simulink model "recovered_model"  (R2024b)
settings: Solver=VariableStepAuto  StartTime=0.0  StopTime=10.0  RelTol=1e-3
libraries: spsIGBTDiodeLib x4, spsSeriesRLCBranchLib x2, spsDCVoltageSourceLib x1, simulink x1, spsVoltageMeasurementLib x1, spspowerguiLib x1
settings Model: Creator=tiany  LastModifiedBy=tiany

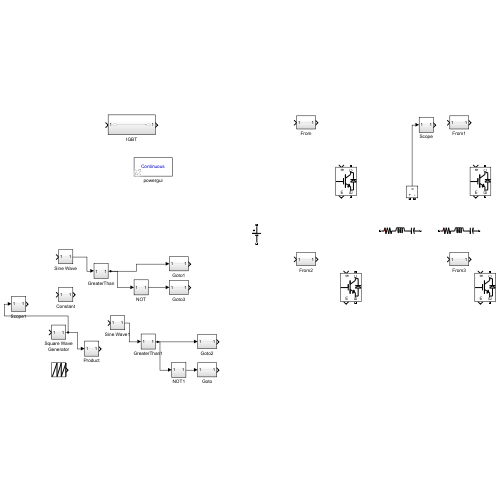
[thumbnail: Simulink's stored preview of the top-level diagram]
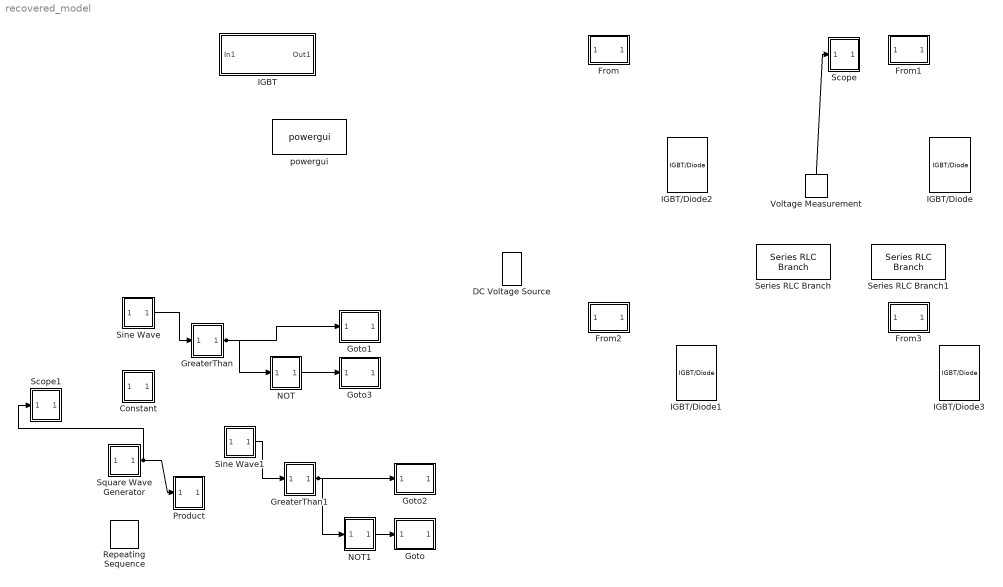
== system recovered_model ==
  Constant : Subsystem
  DC Voltage Source : spsDCVoltageSourceLib/DC Voltage Source  Amplitude=100  Measurements=None
  From : Subsystem
  From1 : Subsystem
  From2 : Subsystem
  From3 : Subsystem
  Goto : Subsystem
  Goto1 : Subsystem
  Goto2 : Subsystem
  Goto3 : Subsystem
  GreaterThan : Subsystem
  GreaterThan1 : Subsystem
  IGBT : Subsystem
  IGBT/Diode{,1..3} (4 alike) : spsIGBTDiodeLib/IGBT//Diode  Ron=1e-3  Rs=1e5  Cs=inf  Measurements=on
  NOT : Subsystem
  NOT1 : Subsystem
  Product : Subsystem
  Repeating Sequence : simulink/Sources/Repeating Sequence  rep_seq_t=[0 2]  rep_seq_y=[0 2]
  Scope : Subsystem
  Scope1 : Subsystem
  Series RLC Branch : spsSeriesRLCBranchLib/Series RLC Branch  LConnTagsString=__new0  RConnTagsString=__new0  BranchType=RLC  Resistance=1  Inductance=1e-3  SetiL0=off  InitialCurrent=0  Capacitance=1e-6  Setx0=off  InitialVoltage=0  Measurements=None
  Series RLC Branch1 : spsSeriesRLCBranchLib/Series RLC Branch  LConnTagsString=__new0  RConnTagsString=__new0  BranchType=RLC  Resistance=1  Inductance=1e-3  SetiL0=off  InitialCurrent=0  Capacitance=1e-6  Setx0=off  InitialVoltage=0  Measurements=None
  Sine Wave : Subsystem
  Sine Wave1 : Subsystem
  Square Wave Generator : Subsystem
  Voltage Measurement : spsVoltageMeasurementLib/Voltage Measurement  PhasorSimulation=off  OutputType=Complex  PSBequivalent=0
  powergui : spspowerguiLib/powergui  Priority=1  SimulationMode=Continuous  SampleTime=50e-6  frequency=60  Iterations=50  frequencyindice=60  Pbase=100e6  ErrMax=1e-4  UnitsV=kV  UnitsW=MW  buscounter=0  FunctionMessages=off  echomessages=off  EnableUseOfTLC=off  CurrentSourceSwitches=off  DisableSnubberDevices=off  DisableRonSwitches=off  DisableVfSwitches=off  DisplayEquations=off  AutomaticDiscreteSolvers=off  SolverType=Tustin/Backward Euler (TBE)  Interpol=off  ExternalGateDelay=off  methode=off  Ts=100  x0status=blocks  SPID=on  SwTol=0  HookPort=off  NonlinearTolerance=1e-4  nMaxIteration=100  ContinueOnMaxIteration=off  RestoreLinks=warning  ResistiveCurrentMeasurement=off  Frange=[0:2:500]  Ylog=off  Xlog=on  ShowGrid=off  save=off  variable=ZData  structure=0  ZoomFFT=off  StartTime=0.0  cycles=1  DisplayStyle=1  fundamental=60  FreqAxis=off  MaxFrequency=1000  frequencyindicesteady=1  RmsSteady=1  display=off
  wires:
  NOT1/1(Out1) -> Goto/1(In1)
  GreaterThan1/1(Out1) -> Goto2/1(In1), NOT1/1(In1)
  Sine Wave1/1(Out1) -> GreaterThan1/1(In1)
  Square Wave Generator/1(Out1) -> Product/1(In1), Scope1/1(In1)
  Voltage Measurement/1 -> Scope/1(In1)
  NOT/1(Out1) -> Goto3/1(In1)
  GreaterThan/1(Out1) -> Goto1/1(In1), NOT/1(In1)
  Sine Wave/1(Out1) -> GreaterThan/1(In1)

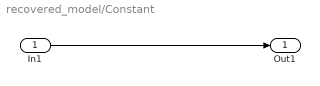
== system recovered_model/Constant ==
  In1 : Inport
  Out1 : Outport
  wires:
  In1/1 -> Out1/1

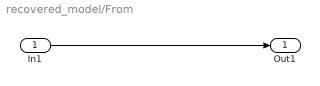
== system recovered_model/From ==
  In1 : Inport
  Out1 : Outport
  wires:
  In1/1 -> Out1/1

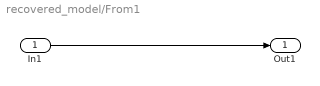
== system recovered_model/From1 ==
  In1 : Inport
  Out1 : Outport
  wires:
  In1/1 -> Out1/1

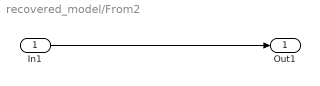
== system recovered_model/From2 ==
  In1 : Inport
  Out1 : Outport
  wires:
  In1/1 -> Out1/1

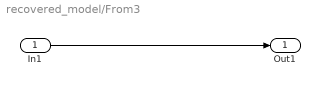
== system recovered_model/From3 ==
  In1 : Inport
  Out1 : Outport
  wires:
  In1/1 -> Out1/1

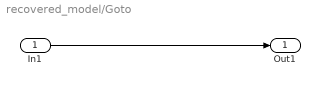
== system recovered_model/Goto ==
  In1 : Inport
  Out1 : Outport
  wires:
  In1/1 -> Out1/1

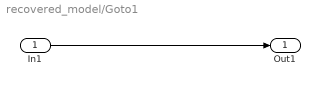
== system recovered_model/Goto1 ==
  In1 : Inport
  Out1 : Outport
  wires:
  In1/1 -> Out1/1

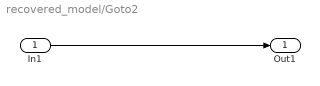
== system recovered_model/Goto2 ==
  In1 : Inport
  Out1 : Outport
  wires:
  In1/1 -> Out1/1

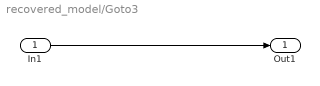
== system recovered_model/Goto3 ==
  In1 : Inport
  Out1 : Outport
  wires:
  In1/1 -> Out1/1

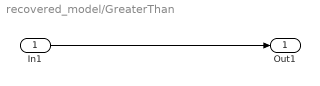
== system recovered_model/GreaterThan ==
  In1 : Inport
  Out1 : Outport
  wires:
  In1/1 -> Out1/1

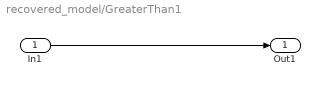
== system recovered_model/GreaterThan1 ==
  In1 : Inport
  Out1 : Outport
  wires:
  In1/1 -> Out1/1

== system recovered_model/IGBT ==
  In1 : Inport
  Out1 : Outport
  wires:
  In1/1 -> Out1/1

== system recovered_model/NOT ==
  In1 : Inport
  Out1 : Outport
  wires:
  In1/1 -> Out1/1

== system recovered_model/NOT1 ==
  In1 : Inport
  Out1 : Outport
  wires:
  In1/1 -> Out1/1

== system recovered_model/Product ==
  In1 : Inport
  Out1 : Outport
  wires:
  In1/1 -> Out1/1

== system recovered_model/Scope ==
  In1 : Inport
  Out1 : Outport
  wires:
  In1/1 -> Out1/1

== system recovered_model/Scope1 ==
  In1 : Inport
  Out1 : Outport
  wires:
  In1/1 -> Out1/1

== system recovered_model/Sine Wave ==
  In1 : Inport
  Out1 : Outport
  wires:
  In1/1 -> Out1/1

== system recovered_model/Sine Wave1 ==
  In1 : Inport
  Out1 : Outport
  wires:
  In1/1 -> Out1/1

== system recovered_model/Square Wave Generator ==
  In1 : Inport
  Out1 : Outport
  wires:
  In1/1 -> Out1/1
